simulink model "QuarterCarModel_nonLin_vs_Lin"  (R2019b)
settings: Solver=FixedStepAuto  StartTime=0.0  StopTime=t_tot  FixedStep=dt  RelTol=1e-3
values from neighbouring files (symbols this model uses):
  A = [0 0 1 0; 0 0 0 1; 0 a_32  0 a_34; a_41 a_42 0 a_44]    [QuarterCarModel.m]
  B = [0; 0; 0; -kt/mu]    [QuarterCarModel.m]
  C = [0 -k/ms 0 -c_min/ms]    [QuarterCarModel.m]
  c_min = 800    [QuarterCarModel.m]
  er = 0.7    [QuarterCarModel.m]
  k = 27000    [QuarterCarModel.m]
  k0 = 38000    [QuarterCarModel.m]
  kt = 300000    [QuarterCarModel.m]
  ms = 450    [QuarterCarModel.m]
  mu = 70    [QuarterCarModel.m]
  uMR = 0    [QuarterCarModel.m]    (also in max_x.m = uMR_values(i))
  wr = 2*pi*v/lc    (= 7.85398163397)    [QuarterCarModel.m]
libraries: simulink x1
settings Model: Creator=Elia  LastModifiedBy=Elia

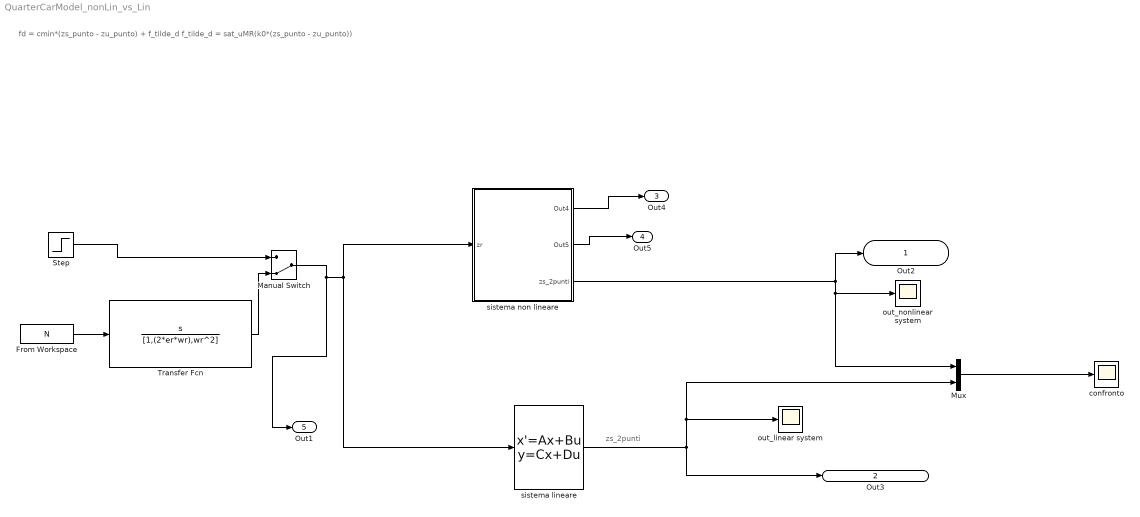
== system QuarterCarModel_nonLin_vs_Lin ==
  note: zs_2punti
  note: fd = cmin*(zs_punto - zu_punto) + f_tilde_d
      |
      | f_tilde_d = sat_uMR(k0*(zs_punto - zu_punto))
  From Workspace : FromWorkspace  VariableName=N  SampleTime=0
  Manual Switch : ManualSwitch  CurrentSetting=0
  Mux : Mux  Inputs=2
  Step : Step  SampleTime=0
  Transfer Fcn : TransferFcn  Numerator=[1,0]  Denominator=[1,(2*er*wr),wr^2]
  confronto : Scope
  out_linear system : Scope
  out_nonlinear system : Scope
  sistema lineare : StateSpace  A=A  B=B  C=C  D=0  InitialCondition=0
  sistema non lineare : Subsystem
  Out2 : Outport  SignalName=zs_2punti_nl
  Out3 : Outport  Port=2  SignalName=zs_2punti_l
  Out4 : Outport  Port=3  SignalName=fd
  Out5 : Outport  Port=4  SignalName=zTilde_punto
  Out1 : Outport  Port=5  SignalName=zr
  wires:
  From Workspace/1 -> Transfer Fcn/1
  sistema lineare/1 -> out_linear system/1, Mux/2, Out3/1
  Mux/1 -> confronto/1
  sistema non lineare/1(Out4) -> Out4/1
  sistema non lineare/2(Out5) -> Out5/1
  sistema non lineare/3(zs_2punti) -> Mux/1, out_nonlinear system/1, Out2/1
  Manual Switch/1 -> Out1/1, sistema lineare/1, sistema non lineare/1(zr)
  Transfer Fcn/1 -> Manual Switch/2
  Step/1 -> Manual Switch/1

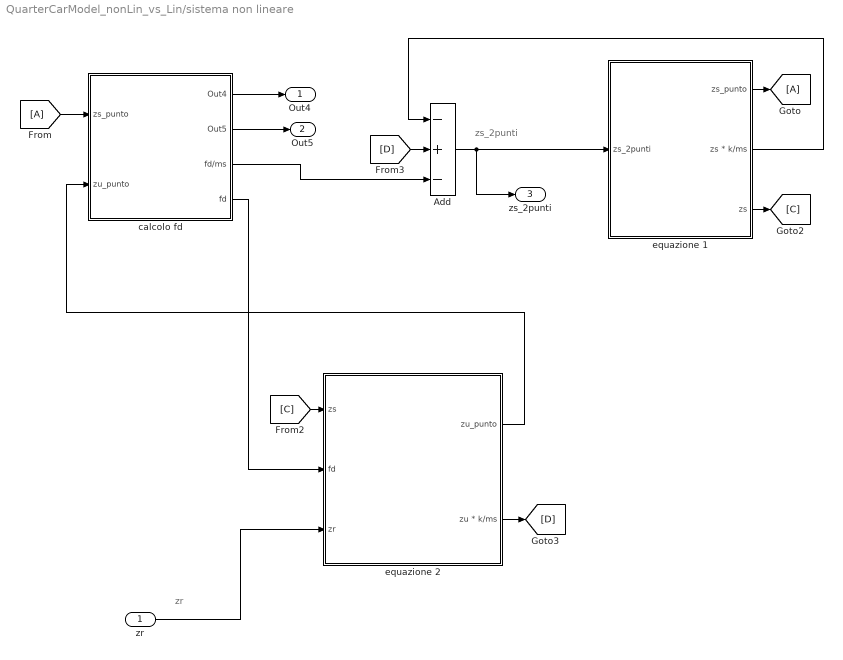
== system QuarterCarModel_nonLin_vs_Lin/sistema non lineare ==
  note: zs_2punti
  note: zr
  zr : Inport
  Add : Sum  Inputs=-+-
  calcolo fd : Subsystem
  equazione 1 : Subsystem
  equazione 2 : Subsystem
  Out4 : Outport
  Out5 : Outport  Port=2
  zs_2punti : Outport  Port=3
  wires:
  calcolo fd/4(fd) -> equazione 2/2(fd)
  equazione 1/3(zs) -> [C]
  calcolo fd/1(Out4) -> Out4/1
  Add/1 -> zs_2punti/1, equazione 1/1(zs_2punti)
  equazione 2/1(zu_punto) -> calcolo fd/2(zu_punto)
  equazione 1/1(zs_punto) -> [A]
  calcolo fd/2(Out5) -> Out5/1
  calcolo fd/3(fd/ms) -> Add/3
  [C] -> equazione 2/1(zs)
  [D] -> Add/2
  equazione 1/2("zs * k/ms ") -> Add/1
  equazione 2/2("zu * k/ms ") -> [D]
  [A] -> calcolo fd/1(zs_punto)
  zr/1 -> equazione 2/3(zr)

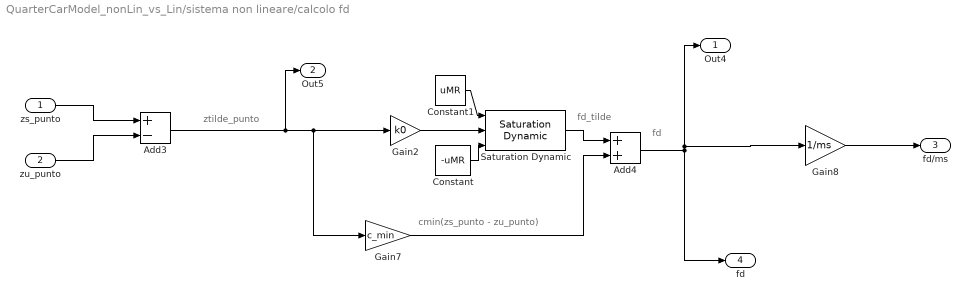
== system QuarterCarModel_nonLin_vs_Lin/sistema non lineare/calcolo fd ==
  note: ztilde_punto
  note: cmin(zs_punto - zu_punto)
  note: fd
  note: fd_tilde
  zs_punto : Inport
  zu_punto : Inport  Port=2
  Add3 : Sum  Inputs=+-
  Add4 : Sum
  Constant : Constant  Value=-uMR
  Constant1 : Constant  Value=uMR
  Gain2 : Gain  Gain=k0
  Gain7 : Gain  Gain=c_min
  Gain8 : Gain  Gain=1/ms
  Saturation Dynamic : simulink/Discontinuities/Saturation Dynamic  OutMin=[]  OutMax=[]  OutDataTypeStr=Inherit: Same as second input  OutDataType=fixdt(1, 16)  OutScaling=2^-10  DoSatur=off
  Out4 : Outport
  Out5 : Outport  Port=2
  fd/ms : Outport  Port=3
  fd : Outport  Port=4
  wires:
  Add3/1 -> Gain2/1, Gain7/1, Out5/1
  Gain2/1 -> Saturation Dynamic/2
  Constant/1 -> Saturation Dynamic/3
  zu_punto/1 -> Add3/2
  Add4/1 -> Gain8/1, Out4/1, fd/1
  Gain8/1 -> fd/ms/1
  Gain7/1 -> Add4/2
  Saturation Dynamic/1 -> Add4/1
  Constant1/1 -> Saturation Dynamic/1
  zs_punto/1 -> Add3/1

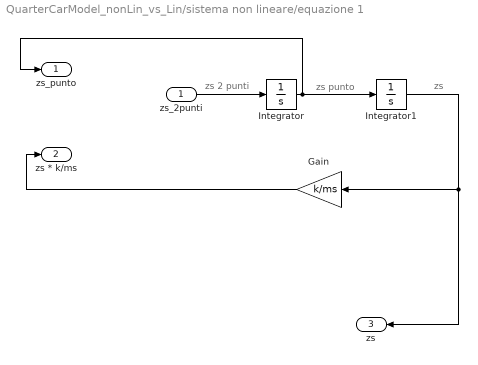
== system QuarterCarModel_nonLin_vs_Lin/sistema non lineare/equazione 1 ==
  note: zs
  note: zs 2 punti
  note: zs punto
  zs_2punti : Inport
  Gain : Gain  Gain=k/ms
  Integrator : Integrator
  Integrator1 : Integrator
  zs_punto : Outport
  "zs * k/ms " : Outport  Port=2
  zs : Outport  Port=3
  wires:
  zs_2punti/1 -> Integrator/1
  Integrator/1 -> zs_punto/1, Integrator1/1
  Integrator1/1 -> zs/1, Gain/1
  Gain/1 -> "zs * k/ms "/1

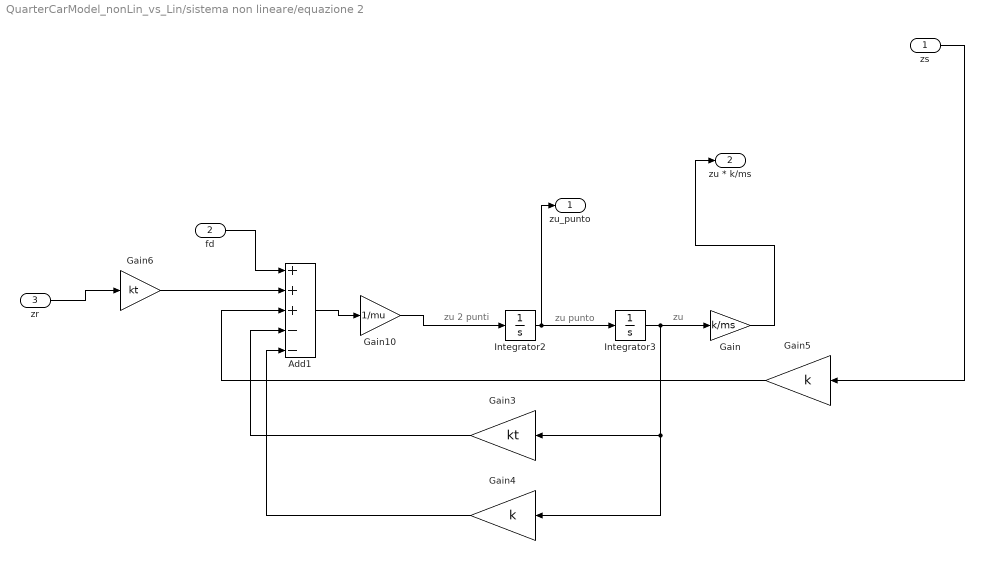
== system QuarterCarModel_nonLin_vs_Lin/sistema non lineare/equazione 2 ==
  note: zu
  note: zu 2 punti
  note: zu punto
  zs : Inport
  fd : Inport  Port=2
  zr : Inport  Port=3
  Add1 : Sum  Inputs=+++--
  Gain : Gain  Gain=k/ms
  Gain10 : Gain  Gain=1/mu
  Gain3 : Gain  Gain=kt
  Gain4 : Gain  Gain=k
  Gain5 : Gain  Gain=k
  Gain6 : Gain  Gain=kt
  Integrator2 : Integrator
  Integrator3 : Integrator
  zu_punto : Outport
  "zu * k/ms " : Outport  Port=2
  wires:
  Integrator2/1 -> zu_punto/1, Integrator3/1
  Integrator3/1 -> Gain3/1, Gain4/1, Gain/1
  Gain6/1 -> Add1/2
  Add1/1 -> Gain10/1
  Gain10/1 -> Integrator2/1
  Gain3/1 -> Add1/4
  Gain5/1 -> Add1/3
  Gain4/1 -> Add1/5
  zr/1 -> Gain6/1
  zs/1 -> Gain5/1
  fd/1 -> Add1/1
  Gain/1 -> "zu * k/ms "/1
